simulink model "Positio_Tracking_Sim"  (R2019a)
settings: Solver=VariableStepAuto  StartTime=0.0  StopTime=10.0  RelTol=1e-3
settings Model: Creator=Karel  LastModifiedBy=Karel

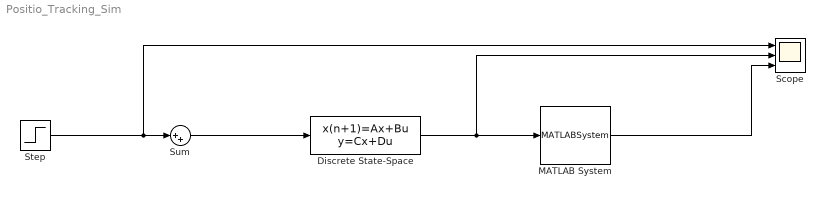
== system Positio_Tracking_Sim ==
  Discrete State-Space : DiscreteStateSpace  SampleTime=-1
  MATLAB System : MATLABSystem
  Scope : Scope  NumInputPorts=3
  Step : Step  SampleTime=0
  Sum : Sum  Inputs=|++
  wires:
  Step/1 -> Sum/1, Scope/1
  Sum/1 -> Discrete State-Space/1
  Discrete State-Space/1 -> Scope/2, MATLAB System/1
  MATLAB System/1 -> Scope/3
